simulink model "Simulink_Fuzzy"  (Simulink 7.1)
settings: Solver=ode45  StartTime=0.0  StopTime=10.0  RelTol=1e-3
values from neighbouring files (symbols this model uses):
  denG = [1 8.876]    [matlab.mat]    (also in workspace.mat)
  numG = 6.39    [matlab.mat]    (also in workspace.mat)
libraries: fuzblock x1
settings Model: Creator=Usuario  LastModifiedBy=Lab Man
settings OptimizationCC: InitFltsAndDblsToZero=off

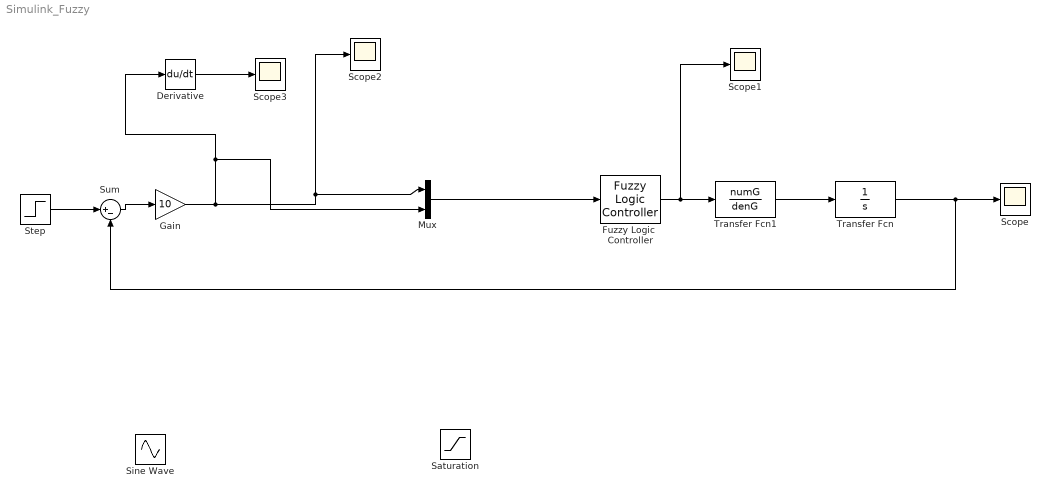
== system Simulink_Fuzzy ==
  Derivative : Derivative
  Fuzzy Logic  Controller : fuzblock/Fuzzy Logic  Controller  SystemSampleTime=-1  fis=FuzzyFinal
  Gain : Gain  Gain=10
  Mux : Mux  Inputs=2
  Saturation : Saturate  UpperLimit=12  LowerLimit=0
  Scope{,1..3} (4 alike) : Scope
      Scope2 settings: SaveName=ScopeData2
      Scope3 settings: SaveName=ScopeData3
  Sine Wave : Sin  SampleTime=0
  Step : Step  Time=0  SampleTime=0
  Sum : Sum  Inputs=|+-
  Transfer Fcn : TransferFcn  Denominator=[1 0]
  Transfer Fcn1 : TransferFcn  Numerator=numG  Denominator=denG
  wires:
  Transfer Fcn1/1 -> Transfer Fcn/1
  Transfer Fcn/1 -> Scope/1, Sum/2
  Gain/1 -> Scope2/1, Mux/1, Derivative/1, Mux/2
  Sum/1 -> Gain/1
  Fuzzy Logic  Controller/1 -> Transfer Fcn1/1, Scope1/1
  Derivative/1 -> Scope3/1
  Mux/1 -> Fuzzy Logic  Controller/1
  Step/1 -> Sum/1
